simulink model "M182_Lab8"  (R2019b)
settings: Solver=VariableStepAuto  StartTime=0.0  StopTime=10.0  RelTol=1e-3
settings Model: Creator=scjcb  LastModifiedBy=scjcb

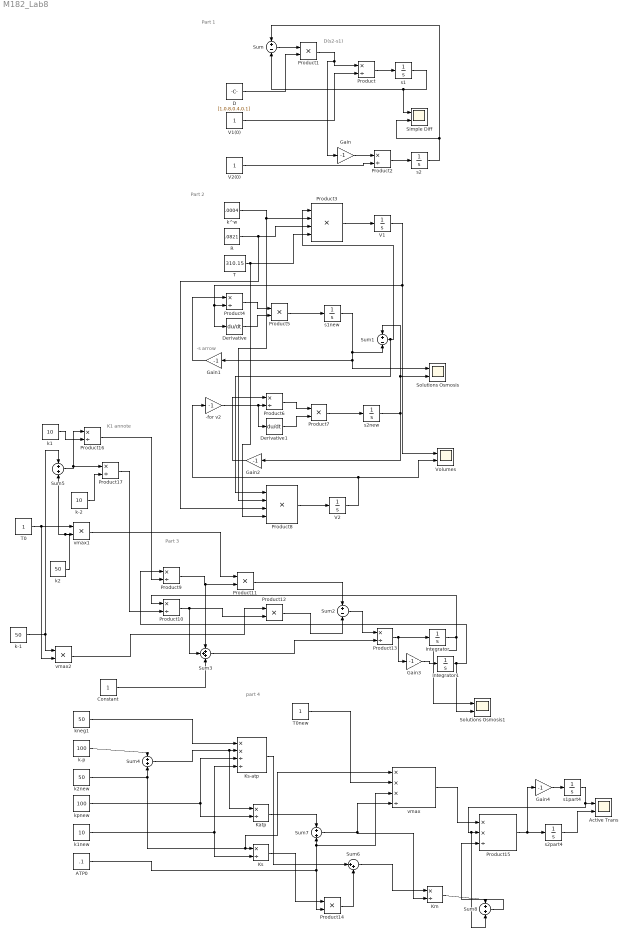
== system M182_Lab8 ==
  note: part 4
  note: K1 annote
  note: Part 3
  note: -s arrow
  note: Part 2
  note: Part 1
  note: D(s2-s1)
  -for v2 : Gain  Gain=-1
  ATP0 : Constant  Value=.1
  Active Trans : Scope  NumInputPorts=2
  Constant : Constant
  D : Constant  Value=[1,0.8,0.4,0.1]
  Derivative : Derivative
  Derivative1 : Derivative
  Gain{,1..4} (5 alike) : Gain  Gain=-1
  Integrator : Integrator  InitialCondition=20
  Integrator1 : Integrator  InitialCondition=80
  Katp : Product  Inputs=*/
  Km : Product  Inputs=*/
  Ks : Product  Inputs=*/
  Ks-atp : Product  Inputs=**//
  Product{,2,4,6,9..10,13,16..17} (9 alike) : Product  Inputs=*/
  Product{1,5,7,14} (4 alike) : Product
  Product11 : Product  Inputs=**
  Product12 : Product  Inputs=**
  Product15 : Product  Inputs=**/
  Product3 : Product  Inputs=****
  Product8 : Product  Inputs=****
  R : Constant  Value=.0821
  Simple Diff : Scope  NumInputPorts=2
  Solutions Osmosis : Scope  NumInputPorts=2
  Solutions Osmosis1 : Scope  NumInputPorts=2
  Sum : Sum  Inputs=+-
  Sum1 : Sum  Inputs=+-
  Sum2 : Sum  Inputs=+-
  Sum3 : Sum  Inputs=+++
  Sum4 : Sum
  Sum5 : Sum
  Sum6 : Sum  Inputs=|++
  Sum7 : Sum
  Sum8 : Sum  Inputs=2
  T : Constant  Value=310.15
  T0 : Constant
  T0new : Constant
  V1 : Integrator  InitialCondition=10
  V1(0) : Constant
  V2 : Integrator  InitialCondition=1
  V2(0) : Constant
  Volumes : Scope  NumInputPorts=2
  k-1 : Constant  Value=50
  k-2 : Constant  Value=10
  k-p : Constant  Value=100
  k1 : Constant  Value=10
  k1new : Constant  Value=10
  k2 : Constant  Value=50
  k2new : Constant  Value=50
  k^w : Constant  Value=.0004
  kneg1 : Constant  Value=50
  kpnew : Constant  Value=100
  s1 : Integrator  InitialCondition=20
  s1new : Integrator
  s1part4 : Integrator  InitialCondition=20
  s2 : Integrator  InitialCondition=80
  s2new : Integrator  InitialCondition=100
  s2part4 : Integrator  InitialCondition=80
  vmax : Product  Inputs=***/
  vmax1 : Product
  vmax2 : Product
  wires:
  s2/1 -> Sum/1, Simple Diff/2
  Sum/1 -> Product1/1
  D/1 -> Product1/2
  V1(0)/1 -> Product/2
  Product1/1 -> Product/1, Gain/1
  Product/1 -> s1/1
  s1/1 -> Simple Diff/1, Sum/2
  V2(0)/1 -> Product2/2
  Gain/1 -> Product2/1
  Product2/1 -> s2/1
  k^w/1 -> Product8/2, Product3/2
  R/1 -> Product8/3, Product3/3
  T/1 -> Product3/4, Product8/4
  Product3/1 -> V1/1
  V1/1 -> Volumes/1, Derivative/1, Product4/2
  s1new/1 -> Gain1/1, Solutions Osmosis/1, Sum1/2
  Gain1/1 -> Product4/1
  Product4/1 -> Product5/1
  Derivative/1 -> Product5/2
  Product5/1 -> s1new/1
  Product7/1 -> s2new/1
  Gain2/1 -> Product6/1
  Derivative1/1 -> Product7/2
  Product6/1 -> Product7/1
  s2new/1 -> Solutions Osmosis/2, Sum1/1, Gain2/1
  -for v2/1 -> Derivative1/1, Product6/2
  Sum1/1 -> Product8/1, Product3/1
  Product8/1 -> V2/1
  V2/1 -> Volumes/2, -for v2/1
  k2/1 -> Sum5/2, vmax1/2
  Product9/1 -> Sum3/1, Product11/2
  Product10/1 -> Sum3/2, Product12/2
  Product11/1 -> Sum2/1
  Product12/1 -> Sum2/2
  Constant/1 -> Sum3/3
  Sum3/1 -> Product13/2
  Sum2/1 -> Product13/1
  Product13/1 -> Gain3/1, Integrator/1
  Gain3/1 -> Integrator1/1
  Integrator1/1 -> Solutions Osmosis1/2, Product9/1
  Integrator/1 -> Solutions Osmosis1/1, Product10/1
  T0/1 -> vmax1/1, vmax2/2
  k-1/1 -> Sum5/1, vmax2/1
  vmax1/1 -> Product11/1
  vmax2/1 -> Product12/1
  Sum5/1 -> Product17/1, Product16/1
  k1/1 -> Product16/2
  Product16/1 -> Product9/2
  k-2/1 -> Product17/2
  Product17/1 -> Product10/2
  k-p/1 -> Sum4/1
  k2new/1 -> vmax/1, Ks/1, Sum4/2
  Sum4/1 -> Katp/1, Ks-atp/2
  kneg1/1 -> Ks-atp/1
  k1new/1 -> Ks/2, Ks-atp/4
  kpnew/1 -> Katp/2, Ks-atp/3
  Katp/1 -> Sum7/1
  ATP0/1 -> Product14/2, vmax/3, Sum7/2
  Sum7/1 -> Km/2, vmax/4
  T0new/1 -> vmax/2
  Ks-atp/1 -> Sum6/1
  Ks/1 -> Product14/1
  Product14/1 -> Sum6/2
  Sum6/1 -> Km/1
  Km/1 -> Sum8/1
  vmax/1 -> Product15/1
  s2part4/1 -> Active Trans/2
  Sum8/1 -> Product15/3
  Product15/1 -> Gain4/1, s2part4/1
  Gain4/1 -> s1part4/1
  s1part4/1 -> Sum8/2, Product15/2, Active Trans/1
